simulink model "coffeeMachine"  (R2020b)
settings: Solver=VariableStepAuto  StartTime=0.0  StopTime=10.0  RelTol=1e-3
undefined symbols (not defined in the file): densAir
libraries: dspnetwork x1
settings Model: Creator=xinbo  LastModifiedBy=xinbo

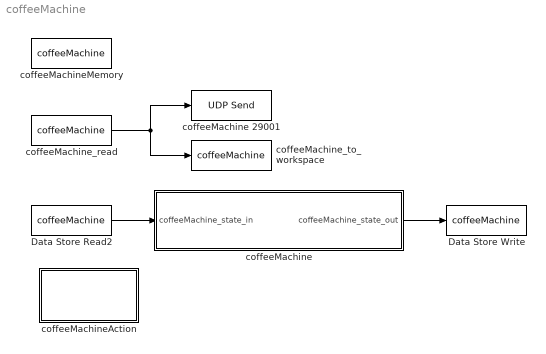
== system coffeeMachine ==
  Data Store Read2 : DataStoreRead  DataStoreName=coffeeMachine
  Data Store Write : DataStoreWrite  DataStoreName=coffeeMachine
  coffeeMachine : Stateflow chart  TreatAsAtomicUnit=on
  coffeeMachine 29001 : dspnetwork/UDP Send  remoteURL='127.0.0.1'  remotePort=29001  localURL='0.0.0.0'  localPortSource=Automatically determine  localPort=-1  sendBufferSize=8192  sampletime=-1  blockPlatform=[]  separateLengthPort=0
  coffeeMachineAction : Subsystem
  coffeeMachineMemory : DataStoreMemory  DataStoreName=coffeeMachine  ReadBeforeWriteMsg=warning  WriteAfterWriteMsg=warning  WriteAfterReadMsg=warning  ShowAdditionalParam=off
  coffeeMachine_read : DataStoreRead  DataStoreName=coffeeMachine
  coffeeMachine_to_workspace : ToWorkspace  VariableName=coffeeMachine  SaveFormat=Timeseries  SampleTime=-1
  wires:
  Data Store Read2/1 -> coffeeMachine/1(coffeeMachine_state_in)
  coffeeMachine_read/1 -> coffeeMachine_to_workspace/1, coffeeMachine 29001/1
  coffeeMachine/1(coffeeMachine_state_out) -> Data Store Write/1

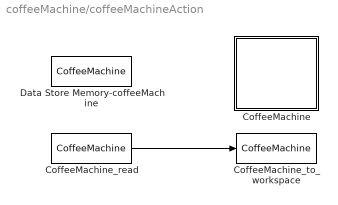
== system coffeeMachine/coffeeMachineAction ==
  CoffeeMachine : Subsystem
      mask Display: image('$imagefile'); % Use "Edit Image" on toolstrip to change.
  CoffeeMachine_read : DataStoreRead  DataStoreName=CoffeeMachine
  CoffeeMachine_to_workspace : ToWorkspace  VariableName=CoffeeMachine  SampleTime=-1
      settings: Save2DSignal=2-D array (concatenate along first dimension)
  Data Store Memory-coffeeMachine : DataStoreMemory  DataStoreName=CoffeeMachine  ReadBeforeWriteMsg=warning  WriteAfterWriteMsg=warning  WriteAfterReadMsg=warning  ShowAdditionalParam=off
  wires:
  CoffeeMachine_read/1 -> CoffeeMachine_to_workspace/1

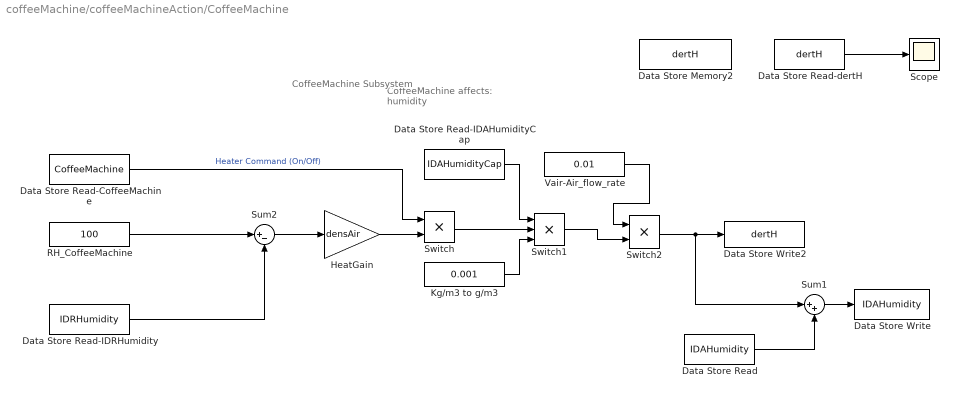
== system coffeeMachine/coffeeMachineAction/CoffeeMachine ==
  note: CoffeeMachine affects:
      | humidity
  note: CoffeeMachine
      |  Subsystem
  " Switch" : Product  RndMeth=Zero
  " Switch1" : Product  Inputs=3  RndMeth=Zero
  " Switch2" : Product  RndMeth=Zero
  Data Store Read : DataStoreRead  DataStoreName=IDAHumidity
  Data Store Read-CoffeeMachine : DataStoreRead  DataStoreName=CoffeeMachine
  Data Store Read-IDAHumidityCap : DataStoreRead  DataStoreName=IDAHumidityCap
  Data Store Read-IDRHumidity : DataStoreRead  DataStoreName=IDRHumidity
  Data Store Read-dertH : DataStoreRead  DataStoreName=dertH
  Data Store Write : DataStoreWrite  DataStoreName=IDAHumidity
  Data Store Write2 : DataStoreWrite  DataStoreName=dertH
  Data Store Memory2 : DataStoreMemory  DataStoreName=dertH  ReadBeforeWriteMsg=warning  WriteAfterWriteMsg=warning  WriteAfterReadMsg=warning  ShowAdditionalParam=off
  HeatGain : Gain  Gain=densAir
  Kg/m3 to g/m3 : Constant  Value=0.001
  RH_CoffeeMachine : Constant  Value=100
  Scope : Scope
  Sum1 : Sum  Inputs=|++
  Sum2 : Sum  Inputs=|+-
  Vair-Air_flow_rate : Constant  Value=0.01
  wires:
  Data Store Read-CoffeeMachine/1 -> " Switch"/1  "Heater Command (On/Off)"
  Sum2/1 -> HeatGain/1
  RH_CoffeeMachine/1 -> Sum2/1
  HeatGain/1 -> " Switch"/2
  " Switch"/1 -> " Switch1"/2
  Data Store Read-IDRHumidity/1 -> Sum2/2
  Data Store Read-IDAHumidityCap/1 -> " Switch1"/1
  Kg/m3 to g/m3/1 -> " Switch1"/3
  " Switch1"/1 -> " Switch2"/2
  Vair-Air_flow_rate/1 -> " Switch2"/1
  " Switch2"/1 -> Sum1/1, Data Store Write2/1
  Sum1/1 -> Data Store Write/1
  Data Store Read-dertH/1 -> Scope/1
  Data Store Read/1 -> Sum1/2

== stateflow chart coffeeMachine/coffeeMachine ==
  state Off
    coffeeMachine_state_out = 0;
  state On
    coffeeMachine_state_out = 1;
  (default) -> Off
  Off -> On : [coffeeMachine_state_in == 1]
  On -> Off : [coffeeMachine_state_in == 0]
  data: coffeeMachine_state_in input; coffeeMachine_state_out output
